simulink model "lab3_car2"  (R2022b)
settings: Solver=VariableStepAuto  StartTime=0.0  StopTime=30  RelTol=1e-3
libraries: simulink x1
settings Model: Creator=khrip  LastModifiedBy=mluser
settings ModelReferenceCC: EnableRefExpFcnMdlSchedulingChecks=on

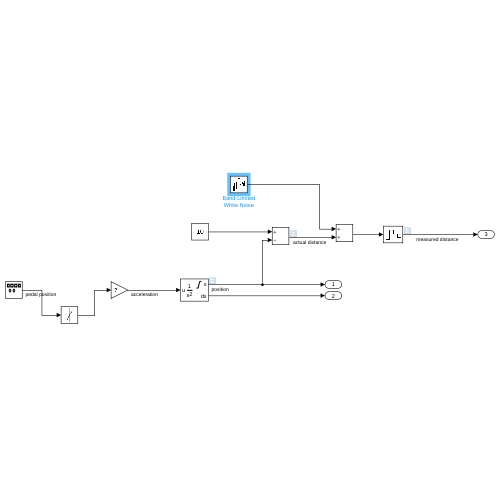
[thumbnail: Simulink's stored preview of the top-level diagram]
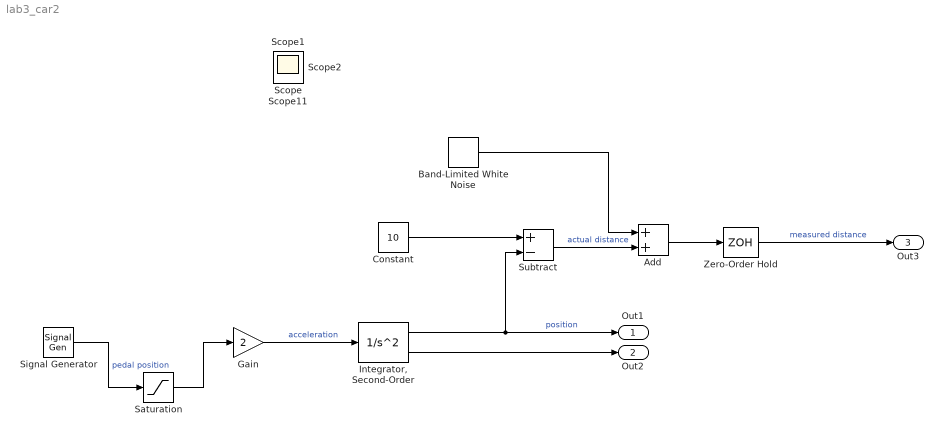
== system lab3_car2 ==
  Add : Sum
  Band-Limited White Noise : simulink/Sources/Band-Limited White Noise  Cov=[0.001]  Ts=0.1  seed=[23341]
  Constant : Constant  Value=10
  Gain : Gain  Gain=2
  "Integrator, Second-Order" : SecondOrderIntegrator  ICX=0  LimitX=on  UpperLimitX=10
  Saturation : Saturate  UpperLimit=inf  LowerLimit=0
  Signal Generator : SignalGenerator  WaveForm=square  Units=rad/sec
  Subtract : Sum  Inputs=+-
  Zero-Order Hold : ZeroOrderHold  SampleTime=0.1
  Out1 : Outport
  Out2 : Outport  Port=2
  Out3 : Outport  Port=3
  Scope{,1..2,11} (4 alike) : Scope
  wires:
  Gain/1 -> "Integrator, Second-Order"/1  "acceleration"
  "Integrator, Second-Order"/1 -> Subtract/2, Out1/1  "position"
  "Integrator, Second-Order"/2 -> Out2/1
  Signal Generator/1 -> Saturation/1  "pedal position"
  Band-Limited White Noise/1 -> Add/1
  Constant/1 -> Subtract/1
  Subtract/1 -> Add/2  "actual distance"
  Add/1 -> Zero-Order Hold/1
  Zero-Order Hold/1 -> Out3/1  "measured distance"
  Saturation/1 -> Gain/1
